simulink model "chap03_25"  (R2021a)
settings: Solver=FixedStepDiscrete  StartTime=0.0  StopTime=7.5  FixedStep=0.001  RelTol=1e-3
undefined symbols (not defined in the file): DiscIntNeverNeededParam
(part 2 of 2)

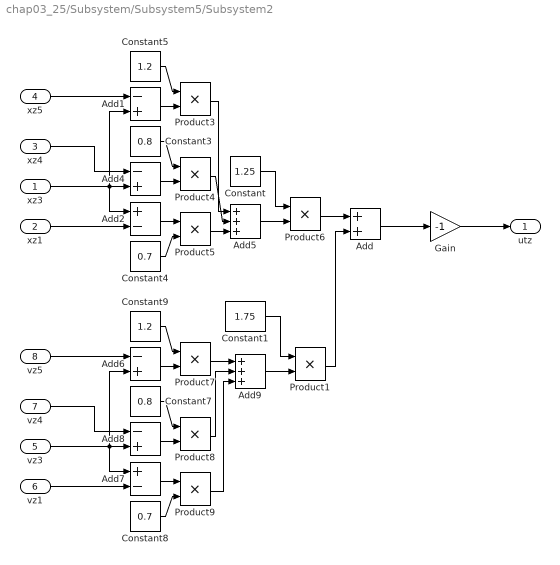
== system chap03_25/Subsystem/Subsystem5/Subsystem2 ==
  xz3 : Inport
  xz1 : Inport  Port=2
  xz4 : Inport  Port=3
  xz5 : Inport  Port=4
  vz3 : Inport  Port=5
  vz1 : Inport  Port=6
  vz4 : Inport  Port=7
  vz5 : Inport  Port=8
  Add : Sum
  Add{1,4,6,8} (4 alike) : Sum  Inputs=-+
  Add2 : Sum  Inputs=+-
  Add5 : Sum  Inputs=+++
  Add7 : Sum  Inputs=+-
  Add9 : Sum  Inputs=+++
  Constant : Constant  Value=1.25
  Constant1 : Constant  Value=1.75
  Constant3 : Constant  Value=0.8
  Constant4 : Constant  Value=0.7
  Constant5 : Constant  Value=1.2
  Constant7 : Constant  Value=0.8
  Constant8 : Constant  Value=0.7
  Constant9 : Constant  Value=1.2
  Gain : Gain  Gain=-1
  Product{1,3..9} (8 alike) : Product
  utz : Outport
  wires:
  Add9/1 -> Product1/2
  Product4/1 -> Add5/2
  Product5/1 -> Add5/3
  Constant3/1 -> Product4/1
  Add4/1 -> Product4/2
  xz3/1 -> Add1/2, Add4/2, Add2/1
  Constant4/1 -> Product5/2
  Product6/1 -> Add/1
  Constant/1 -> Product6/1
  Constant1/1 -> Product1/1
  Product1/1 -> Add/2
  Add2/1 -> Product5/1
  Add5/1 -> Product6/2
  xz4/1 -> Add4/1
  xz1/1 -> Add2/2
  xz5/1 -> Add1/1
  Constant5/1 -> Product3/1
  Add1/1 -> Product3/2
  Product3/1 -> Add5/1
  Product7/1 -> Add9/1
  Add6/1 -> Product7/2
  Constant9/1 -> Product7/1
  vz5/1 -> Add6/1
  vz1/1 -> Add7/2
  vz4/1 -> Add8/1
  Add7/1 -> Product9/1
  Constant8/1 -> Product9/2
  vz3/1 -> Add7/1, Add8/2, Add6/2
  Add8/1 -> Product8/2
  Constant7/1 -> Product8/1
  Product9/1 -> Add9/3
  Product8/1 -> Add9/2
  Gain/1 -> utz/1
  Add/1 -> Gain/1

== system chap03_25/Subsystem/Subsystem5/Subsystem6 ==
  xx3 : Inport
  xx1 : Inport  Port=2
  xx4 : Inport  Port=3
  xx5 : Inport  Port=4
  vx3 : Inport  Port=5
  vx1 : Inport  Port=6
  vx4 : Inport  Port=7
  vx5 : Inport  Port=8
  Add : Sum
  Add{1,4,6,8} (4 alike) : Sum  Inputs=-+
  Add2 : Sum  Inputs=+-
  Add5 : Sum  Inputs=+++
  Add7 : Sum  Inputs=+-
  Add9 : Sum  Inputs=+++
  Constant : Constant  Value=1.25
  Constant1 : Constant  Value=1.75
  Constant3 : Constant  Value=0.8
  Constant4 : Constant  Value=0.7
  Constant5 : Constant  Value=1.2
  Constant7 : Constant  Value=0.8
  Constant8 : Constant  Value=0.7
  Constant9 : Constant  Value=1.2
  Gain : Gain  Gain=-1
  Product{1,3..9} (8 alike) : Product
  utx : Outport
  wires:
  Add9/1 -> Product1/2
  Product4/1 -> Add5/2
  Product5/1 -> Add5/3
  Constant3/1 -> Product4/1
  Add4/1 -> Product4/2
  xx3/1 -> Add1/2, Add4/2, Add2/1
  Constant4/1 -> Product5/2
  Product6/1 -> Add/1
  Constant/1 -> Product6/1
  Constant1/1 -> Product1/1
  Product1/1 -> Add/2
  Add2/1 -> Product5/1
  Add5/1 -> Product6/2
  xx4/1 -> Add4/1
  xx1/1 -> Add2/2
  xx5/1 -> Add1/1
  Constant5/1 -> Product3/1
  Add1/1 -> Product3/2
  Product3/1 -> Add5/1
  Product7/1 -> Add9/1
  Add6/1 -> Product7/2
  Constant9/1 -> Product7/1
  vx5/1 -> Add6/1
  vx1/1 -> Add7/2
  vx4/1 -> Add8/1
  Add7/1 -> Product9/1
  Constant8/1 -> Product9/2
  vx3/1 -> Add7/1, Add8/2, Add6/2
  Add8/1 -> Product8/2
  Constant7/1 -> Product8/1
  Product9/1 -> Add9/3
  Product8/1 -> Add9/2
  Gain/1 -> utx/1
  Add/1 -> Gain/1
